simulink model "integrator_ext_reset_test"  (Simulink 8.7)
settings: Solver=ode45  StartTime=0.0  StopTime=10.0  RelTol=1e-3
undefined symbols (not defined in the file or in its folder): DiscIntNeverNeededParam
settings Model: Creator=arnaud  LastModifiedBy=hamza
settings DataIOCC: SaveFormat=Structure  SignalLoggingSaveFormat=ModelDataLogs
settings OptimizationCC: ExpressionDepthLimit=2147483647
settings DebuggingCC: SolverPrmCheckMsg=warning  FcnCallInpInsideContextMsg=UseLocalSettings  StateNameClashWarn=warning
settings GRTTargetCC: CombineOutputUpdateFcns=off  GRTInterface=on
settings ConfigComp: CovSFcnEnable=off

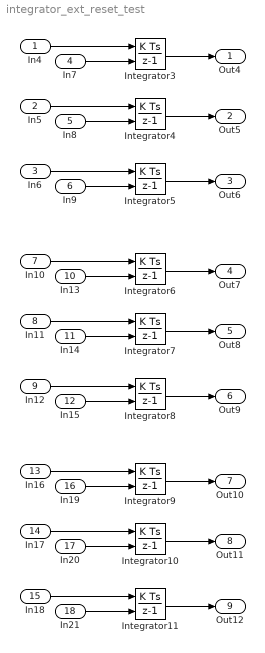
== system integrator_ext_reset_test ==
  In4 : Inport  OutDataTypeStr=double
  In5 : Inport  Port=2  OutDataTypeStr=int32
  In6 : Inport  Port=3  OutDataTypeStr=boolean
  In7 : Inport  Port=4  OutDataTypeStr=double
  In8 : Inport  Port=5  OutDataTypeStr=double
  In9 : Inport  Port=6  OutDataTypeStr=double
  In10 : Inport  Port=7  OutDataTypeStr=double
  In11 : Inport  Port=8  OutDataTypeStr=int32
  In12 : Inport  Port=9  OutDataTypeStr=boolean
  In13 : Inport  Port=10  OutDataTypeStr=int32
  In14 : Inport  Port=11  OutDataTypeStr=int32
  In15 : Inport  Port=12  OutDataTypeStr=int32
  In16 : Inport  Port=13  OutDataTypeStr=double
  In17 : Inport  Port=14  OutDataTypeStr=int32
  In18 : Inport  Port=15  OutDataTypeStr=boolean
  In19 : Inport  Port=16  OutDataTypeStr=boolean
  In20 : Inport  Port=17  OutDataTypeStr=boolean
  In21 : Inport  Port=18  OutDataTypeStr=boolean
  Integrator10 : DiscreteIntegrator  ExternalReset=rising  SampleTime=1.0  ICPrevOutput=DiscIntNeverNeededParam  ICPrevScaledInput=DiscIntNeverNeededParam  mask(DiscretizedDiscreteIntegrator){}
      mask init:
      | %zoh
  Integrator11 : DiscreteIntegrator  ExternalReset=rising  SampleTime=1.0  ICPrevOutput=DiscIntNeverNeededParam  ICPrevScaledInput=DiscIntNeverNeededParam  mask(DiscretizedDiscreteIntegrator){}
      mask init:
      | %zoh
  Integrator3 : DiscreteIntegrator  ExternalReset=rising  SampleTime=1.0  ICPrevOutput=DiscIntNeverNeededParam  ICPrevScaledInput=DiscIntNeverNeededParam  mask(DiscretizedDiscreteIntegrator){}
      mask init:
      | %zoh
  Integrator4 : DiscreteIntegrator  ExternalReset=rising  SampleTime=1.0  ICPrevOutput=DiscIntNeverNeededParam  ICPrevScaledInput=DiscIntNeverNeededParam  mask(DiscretizedDiscreteIntegrator){}
      mask init:
      | %zoh
  Integrator5 : DiscreteIntegrator  ExternalReset=rising  SampleTime=1.0  ICPrevOutput=DiscIntNeverNeededParam  ICPrevScaledInput=DiscIntNeverNeededParam  mask(DiscretizedDiscreteIntegrator){}
      mask init:
      | %zoh
  Integrator6 : DiscreteIntegrator  ExternalReset=rising  SampleTime=1.0  ICPrevOutput=DiscIntNeverNeededParam  ICPrevScaledInput=DiscIntNeverNeededParam  mask(DiscretizedDiscreteIntegrator){}
      mask init:
      | %zoh
  Integrator7 : DiscreteIntegrator  ExternalReset=rising  SampleTime=1.0  ICPrevOutput=DiscIntNeverNeededParam  ICPrevScaledInput=DiscIntNeverNeededParam  mask(DiscretizedDiscreteIntegrator){}
      mask init:
      | %zoh
  Integrator8 : DiscreteIntegrator  ExternalReset=rising  SampleTime=1.0  ICPrevOutput=DiscIntNeverNeededParam  ICPrevScaledInput=DiscIntNeverNeededParam  mask(DiscretizedDiscreteIntegrator){}
      mask init:
      | %zoh
  Integrator9 : DiscreteIntegrator  ExternalReset=rising  SampleTime=1.0  ICPrevOutput=DiscIntNeverNeededParam  ICPrevScaledInput=DiscIntNeverNeededParam  mask(DiscretizedDiscreteIntegrator){}
      mask init:
      | %zoh
  Out4 : Outport
  Out5 : Outport  Port=2
  Out6 : Outport  Port=3
  Out7 : Outport  Port=4
  Out8 : Outport  Port=5
  Out9 : Outport  Port=6
  Out10 : Outport  Port=7
  Out11 : Outport  Port=8
  Out12 : Outport  Port=9
  wires:
  In4/1 -> Integrator3/1
  Integrator3/1 -> Out4/1
  In5/1 -> Integrator4/1
  Integrator4/1 -> Out5/1
  In6/1 -> Integrator5/1
  Integrator5/1 -> Out6/1
  In7/1 -> Integrator3/2
  In8/1 -> Integrator4/2
  In9/1 -> Integrator5/2
  In10/1 -> Integrator6/1
  Integrator6/1 -> Out7/1
  In11/1 -> Integrator7/1
  Integrator7/1 -> Out8/1
  In12/1 -> Integrator8/1
  Integrator8/1 -> Out9/1
  In13/1 -> Integrator6/2
  In14/1 -> Integrator7/2
  In15/1 -> Integrator8/2
  In16/1 -> Integrator9/1
  Integrator9/1 -> Out10/1
  In17/1 -> Integrator10/1
  Integrator10/1 -> Out11/1
  In18/1 -> Integrator11/1
  Integrator11/1 -> Out12/1
  In19/1 -> Integrator9/2
  In20/1 -> Integrator10/2
  In21/1 -> Integrator11/2
